simulink model "Force_Collection"  (Simulink 6.6)
settings: Solver=ode3  StartTime=0.0  StopTime=inf  RelTol=1e-3
StopFcn:
  | %% Name .mat file
  | 
  |     datime = datestr(now);
  |     colon = datime == ':';
  |     space = datime == ' ';
  |     dash  = datime == '-';
  |     datime(colon) = '';
  |     datime(space) = '_';
  |     datime(dash) = '';
  | 
  |     prompt = {'Subject #?','When? (PRE,POST,etc.)','Type of test? (forcepedals)', 'Loaded? (Enter loaded or unloaded)','Trial #? (1,2,...)'};
  | 
  |     dlgTitle = 'File Name';
  |     numlines = 1;
  |     default = {'000','PREPOST','forcepedals','loadedunloaded','1'};
  |     userinfo = inputdlg(prompt,dlgTitle,numlines,default);
  | 
  |     if isempty(userinfo) == 0
  |         sub = userinfo{1};
  |         reltime = userinfo{2};
  |         testype = userinfo{3};
  |         resist  = userinfo{4};
  |         trial   = userinfo{5};
  | 
  |         Filename = strcat('FESCycling_',sub,'_',reltime,'_',testype,'_',resist,'_',trial,'_',datime)
  | 
  | %     cd path_file
  | %
  |         save(Filename)
  |     end
values from neighbouring files (symbols this model uses):
  freq_range = 1022.16    [force_test_load.m]    (also in force_test_load_AnnSavePopup.m = 466.8; force_test_load_orig.m = 466.8; param.m = 865.41)
  freq_zero = -38.15    [force_test_load.m]    (also in force_test_load_AnnSavePopup.m = 116.7756; force_test_load_orig.m = 116.7756; param.m = 39.49)
  slope = 15.81    [force_test_load.m]    (also in force_test_load_AnnSavePopup.m = 14.1374; force_test_load_orig.m = 14.1374; param.m = 14.1374)
undefined symbols (not defined in the file or in its folder): analoginput, parameters
libraries: daqlib x2, ni_lib x1
settings Model: Creator=research  LastModifiedBy=research

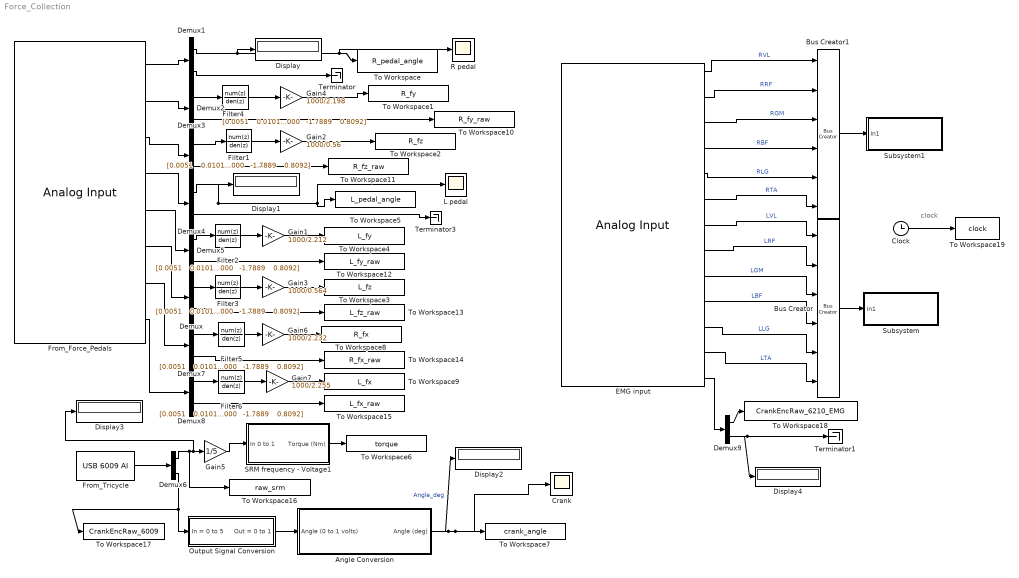
== system Force_Collection ==
  note: clock
  Angle Conversion : Subsystem
  Bus Creator : BusCreator  Inputs=6
  Bus Creator1 : BusCreator  Inputs=6
  Clock : Clock
      settings: Decimation=10
  Crank : Scope
      settings: YMin=0  YMax=375
  Demux{,1..9} (10 alike) : Demux  Outputs=2
  Display{,1..4} (5 alike) : Display
  EMG input : daqlib/Analog Input  DialogController=daqcreatedialog  DialogControllerArgs=DataTag0  AcqMode=0  Device=nidaq Dev3 (USB-6210)  ObjConstructor=analoginput('nidaq','Dev3')  SampleRate=4000  ActualRate=4000  SamplesPerFrame=2  InputType=SingleEnded  NChannelsSelected=13  Channels=1$0$$1$#1$1$$1$#1$2$$1$#1$3$$1$#1$4$$1$#1$5$$1$#1$6$$1$#1$7$$1$#1$8$$1$#1$9$$1$#1$10$$1$#1$11$$1$#1$12$$1$#0$13$$1$#0$14$$1$#0$15$$1$#  NPorts=1 per hardware channel  DataType=double
      settings: SignalType=Sample-based
  Filter{1..6} (6 alike) : DiscreteTransferFcn  Numerator="[0.0051    0.0101    0.0051]"  Denominator="[1.0000   -1.7889    0.8092]"  SampleTime=-1
  From_Force_Pedals : daqlib/Analog Input  DialogController=daqcreatedialog  DialogControllerArgs=DataTag1  AcqMode=0  Device=nidaq Dev1 (DAQCard-6062E)  ObjConstructor=analoginput('nidaq','Dev1')  SampleRate=1000  ActualRate=1000  SamplesPerFrame=2  InputType=Differential  NChannelsSelected=8  Channels=1$0$$1$#1$1$$1$#1$2$$1$#1$3$$1$#1$4$$1$#1$5$$1$#1$6$$1$#1$7$$1$#  NPorts=1 per hardware channel  DataType=double
      settings: SignalType=Sample-based
  From_Tricycle : ni_lib/USB 6009 AI  channels=[1 3]  Ts=0.01  inp_min=-5  inp_max=5  terminalcfg=RSE
  Gain1 : Gain  Gain=1000/2.212
  Gain2 : Gain  Gain=1000/0.56
  Gain3 : Gain  Gain=1000/0.564
  Gain4 : Gain  Gain=1000/2.198
  Gain5 : Gain  Gain=1/5
  Gain6 : Gain  Gain=1000/2.232
  Gain7 : Gain  Gain=1000/2.255
  L pedal : Scope
      settings: YMin=0  YMax=10  SaveName=ScopeData2
  Output Signal Conversion : Subsystem
  R pedal : Scope
      settings: YMin=0  YMax=10
  SRM frequency - Voltage1 : Subsystem
  Subsystem : Subsystem
  Subsystem1 : Subsystem
  Terminator : Terminator
  Terminator1 : Terminator
  Terminator3 : Terminator
  To Workspace : ToWorkspace  VariableName=R_pedal_angle  SampleTime=-1  SaveFormat=Structure With Time
  To Workspace1 : ToWorkspace  VariableName=R_fy  SampleTime=-1  SaveFormat=Structure With Time
  To Workspace10 : ToWorkspace  VariableName=R_fy_raw  SampleTime=-1  SaveFormat=Structure With Time
  To Workspace11 : ToWorkspace  VariableName=R_fz_raw  SampleTime=-1  SaveFormat=Structure With Time
  To Workspace12 : ToWorkspace  VariableName=L_fy_raw  SampleTime=-1  SaveFormat=Structure With Time
  To Workspace13 : ToWorkspace  VariableName=L_fz_raw  SampleTime=-1  SaveFormat=Structure With Time
  To Workspace14 : ToWorkspace  VariableName=R_fx_raw  SampleTime=-1  SaveFormat=Structure With Time
  To Workspace15 : ToWorkspace  VariableName=L_fx_raw  SampleTime=-1  SaveFormat=Structure With Time
  To Workspace16 : ToWorkspace  VariableName=raw_srm  SampleTime=-1  SaveFormat=Structure With Time
  To Workspace17 : ToWorkspace  VariableName=CrankEncRaw_6009  SampleTime=-1  SaveFormat=Structure With Time
  To Workspace18 : ToWorkspace  VariableName=CrankEncRaw_6210_EMG  SampleTime=-1  SaveFormat=Structure
  To Workspace19 : ToWorkspace  VariableName=clock  SampleTime=-1  SaveFormat=Structure
  To Workspace2 : ToWorkspace  VariableName=R_fz  SampleTime=-1  SaveFormat=Structure With Time
  To Workspace3 : ToWorkspace  VariableName=L_fz  SampleTime=-1  SaveFormat=Structure With Time
  To Workspace4 : ToWorkspace  VariableName=L_fy  SampleTime=-1  SaveFormat=Structure With Time
  To Workspace5 : ToWorkspace  VariableName=L_pedal_angle  SampleTime=-1  SaveFormat=Structure With Time
  To Workspace6 : ToWorkspace  VariableName=torque  SampleTime=-1  SaveFormat=Structure With Time
  To Workspace7 : ToWorkspace  VariableName=crank_angle  SampleTime=-1  SaveFormat=Structure With Time
  To Workspace8 : ToWorkspace  VariableName=R_fx  SampleTime=-1  SaveFormat=Structure With Time
  To Workspace9 : ToWorkspace  VariableName=L_fx  SampleTime=-1  SaveFormat=Structure With Time
  wires:
  From_Force_Pedals/1 -> Demux1/1
  Demux1/1 -> Display/1, To Workspace/1, R pedal/1
  Demux1/2 -> Terminator/1
  From_Force_Pedals/2 -> Demux2/1
  Demux2/1 -> Filter4/1
  Demux/1 -> Filter3/1
  From_Force_Pedals/3 -> Demux3/1
  From_Force_Pedals/4 -> Demux4/1
  Demux4/1 -> Display1/1, To Workspace5/1, L pedal/1
  Demux4/2 -> Terminator3/1
  From_Force_Pedals/5 -> Demux5/1
  Demux5/1 -> Filter2/1
  From_Force_Pedals/6 -> Demux/1
  Filter1/1 -> Gain2/1
  Demux3/1 -> Filter1/1
  Gain2/1 -> To Workspace2/1
  Filter3/1 -> Gain3/1
  Gain3/1 -> To Workspace3/1
  Filter2/1 -> Gain1/1
  Gain1/1 -> To Workspace4/1
  Filter4/1 -> Gain4/1
  Gain4/1 -> To Workspace1/1
  Gain5/1 -> SRM frequency - Voltage1/1(In 0 to 1)
  From_Tricycle/1 -> Demux6/1
  Demux6/1 -> To Workspace16/1, Gain5/1, Display3/1
  From_Force_Pedals/8 -> Demux8/1
  From_Force_Pedals/7 -> Demux7/1
  Demux7/1 -> Filter5/1
  Demux8/1 -> Filter6/1
  Filter5/1 -> Gain6/1
  Filter6/1 -> Gain7/1
  Gain6/1 -> To Workspace8/1
  Gain7/1 -> To Workspace9/1
  Demux2/2 -> To Workspace10/1
  Demux3/2 -> To Workspace11/1
  Demux5/2 -> To Workspace12/1
  Demux/2 -> To Workspace13/1
  Demux7/2 -> To Workspace14/1
  Demux8/2 -> To Workspace15/1
  SRM frequency - Voltage1/1(Torque (Nm)) -> To Workspace6/1
  Output Signal Conversion/1(Out = 0 to 1) -> Angle Conversion/1(Angle (0 to 1 volts))
  Demux6/2 -> Output Signal Conversion/1(In = 0 to 5), To Workspace17/1
  Angle Conversion/1(Angle (deg)) -> To Workspace7/1, Crank/1, Display2/1  "Angle_deg"
  EMG input/7 -> Bus Creator/1  "LVL"
  EMG input/1 -> Bus Creator1/1  "RVL"
  EMG input/2 -> Bus Creator1/2  "RRF"
  EMG input/3 -> Bus Creator1/3  "RGM"
  EMG input/4 -> Bus Creator1/4  "RBF"
  EMG input/5 -> Bus Creator1/5  "RLG"
  EMG input/6 -> Bus Creator1/6  "RTA"
  Bus Creator1/1 -> Subsystem1/1(In1)
  EMG input/8 -> Bus Creator/2  "LRF"
  EMG input/9 -> Bus Creator/3  "LGM"
  EMG input/10 -> Bus Creator/4  "LBF"
  EMG input/11 -> Bus Creator/5  "LLG"
  EMG input/12 -> Bus Creator/6  "LTA"
  Bus Creator/1 -> Subsystem/1(In1)
  Clock/1 -> To Workspace19/1
  EMG input/13 -> Demux9/1
  Demux9/1 -> To Workspace18/1
  Demux9/2 -> Terminator1/1, Display4/1

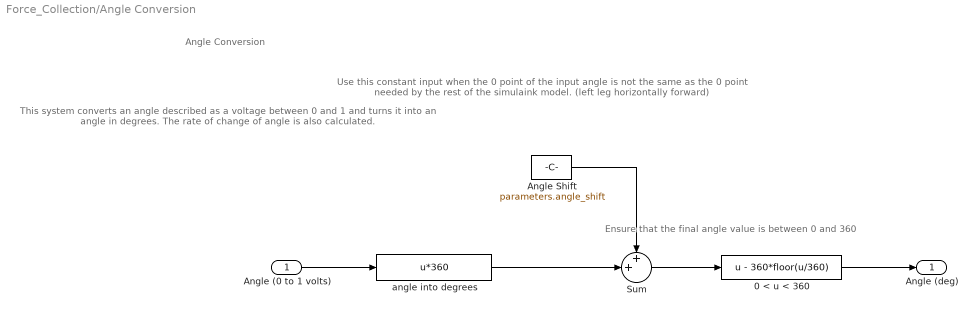
== system Force_Collection/Angle Conversion ==
  note: This system converts an
      | angle described as a voltage
      | between 0 and 1 and turns it
      | into an angle in degrees.
      | The rate of change of angle
      | is also calculated.
  note: Ensure that the final angle
      | value is between 0 and 360
  note: Use this constant input
      | when the 0 point of the
      | input angle is not the same
      | as the 0 point needed by
      | the rest of the simulaink
      | model.
      | (left leg horizontally forward)
  note: Angle Conversion
  Angle (0 to 1 volts) : Inport
  0 < u < 360 : Fcn  Expr=u - 360*floor(u/360)
  Angle Shift : Constant  Value=parameters.angle_shift
  Sum : Sum  Inputs=++|  SaturateOnIntegerOverflow=on  InputSameDT=on
  angle into degrees : Fcn  Expr=u*360
  Angle (deg) : Outport
  wires:
  angle into degrees/1 -> Sum/2
  Sum/1 -> 0 < u < 360/1
  0 < u < 360/1 -> Angle (deg)/1
  Angle (0 to 1 volts)/1 -> angle into degrees/1
  Angle Shift/1 -> Sum/1

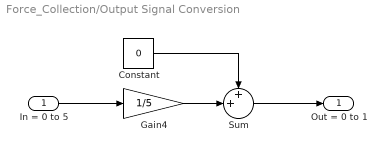
== system Force_Collection/Output Signal Conversion ==
  In = 0 to 5 : Inport
  Constant : Constant  Value=0
  Gain4 : Gain  Gain=1/5  SaturateOnIntegerOverflow=on
  Sum : Sum  Inputs=++|  SaturateOnIntegerOverflow=on  InputSameDT=on
  Out = 0 to 1 : Outport
  wires:
  In = 0 to 5/1 -> Gain4/1
  Sum/1 -> Out = 0 to 1/1
  Constant/1 -> Sum/1
  Gain4/1 -> Sum/2

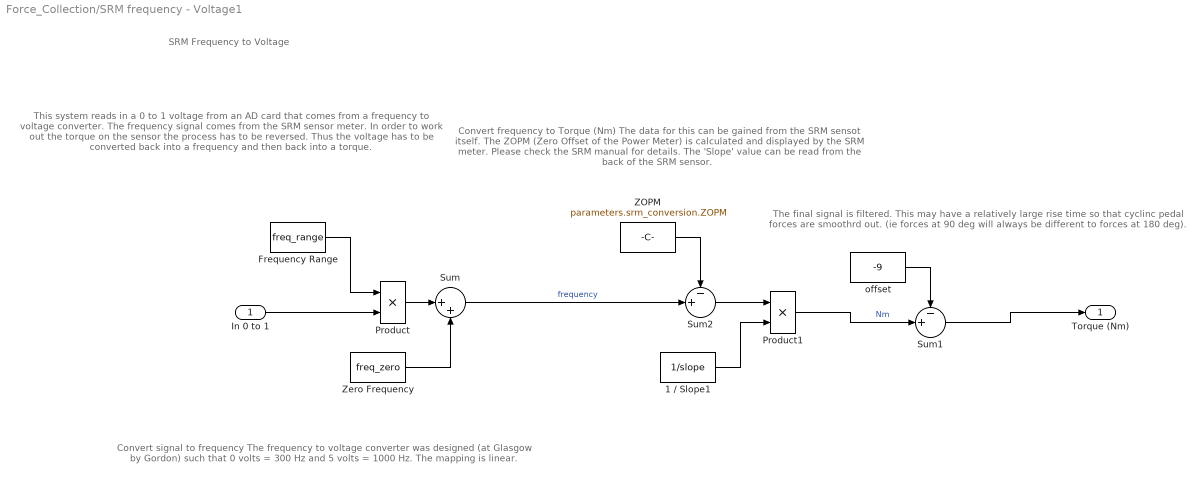
== system Force_Collection/SRM frequency - Voltage1 ==
  note: Convert frequency to Torque (Nm)
      |
      | The data for this can be gained
      | from the SRM sensot itself. The
      | ZOPM (Zero Offset of the Power
      | Meter) is calculated and displayed
      | by the SRM meter.  Please check
      | the SRM manual for details. The
      | 'Slope' value can be read from the
      | back of the SRM sensor.
  note: SRM Frequency to Voltage
  note: This system reads in a 0 to 1 voltage
      | from an AD card that comes from a
      | frequency to voltage converter.  The
      | frequency signal comes from the SRM
      | sensor meter.  In order to work out the
      | torque on the sensor the process has
      | to be reversed.  Thus the voltage has
      | to be converted back into a frequency
      | and then back into a torque.
  note: Convert signal to frequency
      |
      | The frequency to voltage converter
      | was designed (at Glasgow by
      | Gordon) such that 0 volts = 300 Hz
      | and 5 volts = 1000 Hz.  The
      | mapping is linear.
  note: The final signal is filtered.
      | This may have a relatively
      | large rise time so that
      | cyclinc pedal forces are
      | smoothrd out. (ie forces at
      | 90 deg will always be
      | different to forces at 180
      | deg).
  In 0 to 1 : Inport
  1 / Slope1 : Constant  Value=1/slope
  Frequency Range : Constant  Value=freq_range
  Product : Product  SaturateOnIntegerOverflow=on  InputSameDT=on
  Product1 : Product  SaturateOnIntegerOverflow=on  InputSameDT=on
  Sum : Sum  Inputs=|++  SaturateOnIntegerOverflow=on  InputSameDT=on
  Sum1 : Sum  Inputs=-+|  SaturateOnIntegerOverflow=on  InputSameDT=on
  Sum2 : Sum  Inputs=-+|  SaturateOnIntegerOverflow=on  InputSameDT=on
  ZOPM : Constant  Value=parameters.srm_conversion.ZOPM
  Zero Frequency : Constant  Value=freq_zero
  offset : Constant  Value=-9
  Torque (Nm) : Outport
  wires:
  Zero Frequency/1 -> Sum/2
  1 / Slope1/1 -> Product1/2
  ZOPM/1 -> Sum2/1
  Frequency Range/1 -> Product/1
  Sum/1 -> Sum2/2  "frequency"
  In 0 to 1/1 -> Product/2
  Product/1 -> Sum/1
  Sum2/1 -> Product1/1
  Product1/1 -> Sum1/2  "Nm"
  Sum1/1 -> Torque (Nm)/1
  offset/1 -> Sum1/1

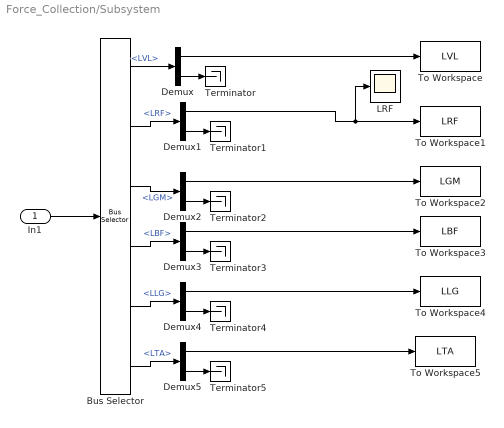
== system Force_Collection/Subsystem ==
  In1 : Inport
  Bus Selector : BusSelector  OutputSignals=LVL,LRF,LGM,LBF,LLG,LTA
  Demux{,1..5} (6 alike) : Demux  Outputs=2
  LRF : Scope
  Terminator{,1..5} (6 alike) : Terminator
  To Workspace : ToWorkspace  VariableName=LVL  SampleTime=-1  SaveFormat=Structure
  To Workspace1 : ToWorkspace  VariableName=LRF  SampleTime=-1  SaveFormat=Structure
  To Workspace2 : ToWorkspace  VariableName=LGM  SampleTime=-1  SaveFormat=Structure
  To Workspace3 : ToWorkspace  VariableName=LBF  SampleTime=-1  SaveFormat=Structure
  To Workspace4 : ToWorkspace  VariableName=LLG  SampleTime=-1  SaveFormat=Structure
  To Workspace5 : ToWorkspace  VariableName=LTA  SampleTime=-1  SaveFormat=Structure
  wires:
  In1/1 -> Bus Selector/1
  Bus Selector/1 -> Demux/1  "<LVL>"
  Demux/2 -> Terminator/1
  Demux/1 -> To Workspace/1
  Demux1/2 -> Terminator1/1
  Demux2/2 -> Terminator2/1
  Demux2/1 -> To Workspace2/1
  Demux3/2 -> Terminator3/1
  Demux4/2 -> Terminator4/1
  Demux5/2 -> Terminator5/1
  Bus Selector/2 -> Demux1/1  "<LRF>"
  Bus Selector/3 -> Demux2/1  "<LGM>"
  Bus Selector/4 -> Demux3/1  "<LBF>"
  Bus Selector/5 -> Demux4/1  "<LLG>"
  Bus Selector/6 -> Demux5/1  "<LTA>"
  Demux1/1 -> To Workspace1/1, LRF/1
  Demux3/1 -> To Workspace3/1
  Demux4/1 -> To Workspace4/1
  Demux5/1 -> To Workspace5/1

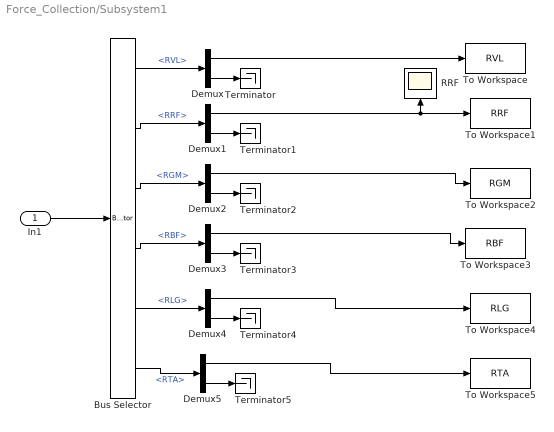
== system Force_Collection/Subsystem1 ==
  In1 : Inport
  Bus Selector : BusSelector  OutputSignals=RVL,RRF,RGM,RBF,RLG,RTA
  Demux{,1..5} (6 alike) : Demux  Outputs=2
  RRF : Scope
      settings: Orientation=up
  Terminator{,1..5} (6 alike) : Terminator
  To Workspace : ToWorkspace  VariableName=RVL  SampleTime=-1  SaveFormat=Structure
  To Workspace1 : ToWorkspace  VariableName=RRF  SampleTime=-1  SaveFormat=Structure
  To Workspace2 : ToWorkspace  VariableName=RGM  SampleTime=-1  SaveFormat=Structure
  To Workspace3 : ToWorkspace  VariableName=RBF  SampleTime=-1  SaveFormat=Structure
  To Workspace4 : ToWorkspace  VariableName=RLG  SampleTime=-1  SaveFormat=Structure
  To Workspace5 : ToWorkspace  VariableName=RTA  SampleTime=-1  SaveFormat=Structure
  wires:
  In1/1 -> Bus Selector/1
  Bus Selector/1 -> Demux/1  "<RVL>"
  Demux/1 -> To Workspace/1
  Demux/2 -> Terminator/1
  Bus Selector/2 -> Demux1/1  "<RRF>"
  Demux1/2 -> Terminator1/1
  Demux1/1 -> To Workspace1/1, RRF/1
  Bus Selector/3 -> Demux2/1  "<RGM>"
  Demux2/2 -> Terminator2/1
  Demux2/1 -> To Workspace2/1
  Bus Selector/4 -> Demux3/1  "<RBF>"
  Demux3/2 -> Terminator3/1
  Demux3/1 -> To Workspace3/1
  Demux4/2 -> Terminator4/1
  Bus Selector/5 -> Demux4/1  "<RLG>"
  Demux4/1 -> To Workspace4/1
  Demux5/2 -> Terminator5/1
  Demux5/1 -> To Workspace5/1
  Bus Selector/6 -> Demux5/1  "<RTA>"
